simulink library "ESPI_lib"  (Simulink 7.5)
settings: Solver=ode45  StartTime=0.0  StopTime=10.0  RelTol=1e-3
values from neighbouring files (symbols this model uses):
  pESPI_bool_AltitudeSel_C = Simulink.Parameter    [ESPI_par.m]
  pESPI_bool_VehSpdDetdEna_C = Simulink.Parameter    [ESPI_par.m]
  pESPI_kmph_MinSpdSnsrThd_C = Simulink.Parameter    [ESPI_par.m]
  pESPI_kmph_SpdThdPlausibiErr_MAP = Simulink.Parameter    [ESPI_par.m]
  pESPI_kPa_VacAmbPres_C = Simulink.Parameter    [ESPI_par.m]
  pESPI_kPa_VacAmbPres_CUR = Simulink.Parameter    [ESPI_par.m]
  pESPI_m_TireDiam_C = Simulink.Parameter    [ESPI_par.m]
  pESPI_mV_VacAmbPres_TAB = Simulink.Parameter    [ESPI_par.m]
  pESPI_Nm_TrqReqZero_C = Simulink.Parameter    [ESPI_par.m]
  pESPI_pct_ABSFact100_C = Simulink.Parameter    [ESPI_par.m]
  pESPI_ratio_ABSFactRateLo_C = Simulink.Parameter    [ESPI_par.m]
  pESPI_ratio_ABSFactRateUp_C = Simulink.Parameter    [ESPI_par.m]
  pESPI_ratio_AltitudeFacDeflt_C = Simulink.Parameter    [ESPI_par.m]
  pESPI_ratio_AltitudeFacMax_C = Simulink.Parameter    [ESPI_par.m]
  pESPI_ratio_AltitudeFacMin_C = Simulink.Parameter    [ESPI_par.m]
  pESPI_ratio_mpsTokmp_C = Simulink.Parameter    [ESPI_par.m]
  pESPI_ratio_TrsmRat_C = Simulink.Parameter    [ESPI_par.m]
  pESPI_s_NoOfSec_C = Simulink.Parameter    [ESPI_par.m]
undefined symbols (not defined in the file or in its folder): p_bool_False_M, p_bool_True_M, p_single_Minus_M, p_single_Zero_M, VehSpdSourceTyp
libraries: BaseOperationLib_Browser x81, PES_CZ_FAW x6, simulink x1
settings Model: Creator=wuaibin  LastModifiedBy=wuaibin

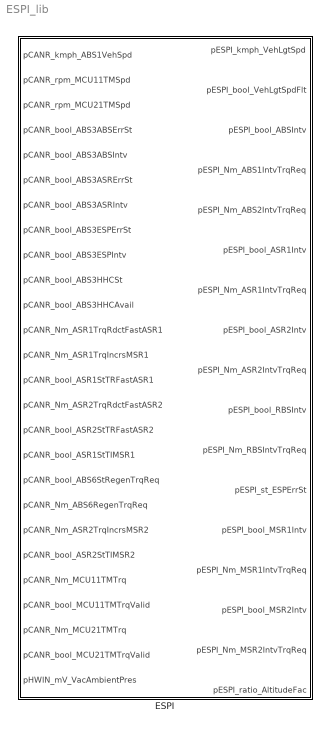
== system ESPI_lib ==
  ESPI : Subsystem  TreatAsAtomicUnit=on

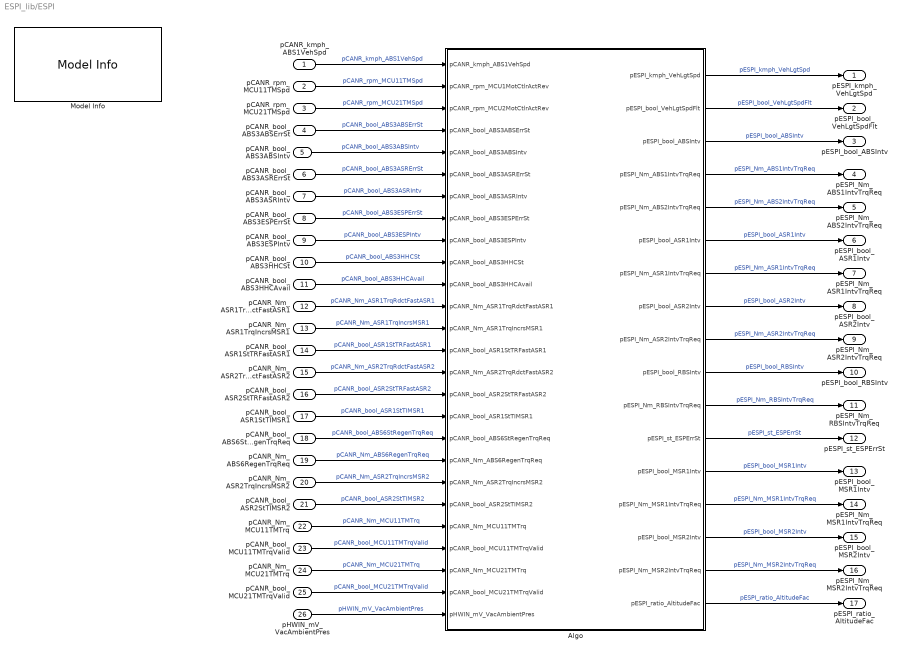
== system ESPI_lib/ESPI ==
  pCANR_kmph_ABS1VehSpd : Inport  OutDataType=fixdt(1, 16)  OutScaling=2^0
  pCANR_rpm_MCU11TMSpd : Inport  Port=2  OutDataType=fixdt(1, 16)  OutScaling=2^0
  pCANR_rpm_MCU21TMSpd : Inport  Port=3  OutDataType=fixdt(1, 16)  OutScaling=2^0
  pCANR_bool_ABS3ABSErrSt : Inport  Port=4  OutDataType=fixdt(1, 16)  OutScaling=2^0
  pCANR_bool_ABS3ABSIntv : Inport  Port=5
  pCANR_bool_ABS3ASRErrSt : Inport  Port=6  OutDataType=fixdt(1, 16)  OutScaling=2^0
  pCANR_bool_ABS3ASRIntv : Inport  Port=7  OutDataType=fixdt(1, 16)  OutScaling=2^0
  pCANR_bool_ABS3ESPErrSt : Inport  Port=8  OutDataType=fixdt(1, 16)  OutScaling=2^0
  pCANR_bool_ABS3ESPIntv : Inport  Port=9  OutDataType=fixdt(1, 16)  OutScaling=2^0
  pCANR_bool_ABS3HHCSt : Inport  Port=10  OutDataType=fixdt(1, 16)  OutScaling=2^0
  pCANR_bool_ABS3HHCAvail : Inport  Port=11  OutDataType=fixdt(1, 16)  OutScaling=2^0
  pCANR_Nm_ASR1TrqRdctFastASR1 : Inport  Port=12  OutDataType=fixdt(1, 16)  OutScaling=2^0
  pCANR_Nm_ASR1TrqIncrsMSR1 : Inport  Port=13  OutDataType=fixdt(1, 16)  OutScaling=2^0
  pCANR_bool_ASR1StTRFastASR1 : Inport  Port=14  OutDataType=fixdt(1, 16)  OutScaling=2^0
  pCANR_Nm_ASR2TrqRdctFastASR2 : Inport  Port=15  OutDataType=fixdt(1, 16)  OutScaling=2^0
  pCANR_bool_ASR2StTRFastASR2 : Inport  Port=16  OutDataType=fixdt(1, 16)  OutScaling=2^0
  pCANR_bool_ASR1StTIMSR1 : Inport  Port=17  OutDataType=fixdt(1, 16)  OutScaling=2^0
  pCANR_bool_ABS6StRegenTrqReq : Inport  Port=18  OutDataType=fixdt(1, 16)  OutScaling=2^0
  pCANR_Nm_ABS6RegenTrqReq : Inport  Port=19  OutDataType=fixdt(1, 16)  OutScaling=2^0
  pCANR_Nm_ASR2TrqIncrsMSR2 : Inport  Port=20  OutDataType=fixdt(1, 16)  OutScaling=2^0
  pCANR_bool_ASR2StTIMSR2 : Inport  Port=21  OutDataType=fixdt(1, 16)  OutScaling=2^0
  pCANR_Nm_MCU11TMTrq : Inport  Port=22
  pCANR_bool_MCU11TMTrqValid : Inport  Port=23
  pCANR_Nm_MCU21TMTrq : Inport  Port=24
  pCANR_bool_MCU21TMTrqValid : Inport  Port=25
  pHWIN_mV_VacAmbientPres : Inport  Port=26
  Algo : Subsystem
  Model Info : simulink/Model-Wide Utilities/Model Info  SystemSampleTime=-1  InitialBlockCM=None  BlockCM=None  Frame=on  DisplayStringWithTags=Model Info\nCreated: %<Created>\nCreator: %<Creator>  HorizontalTextAlignment=Center  LeftAlignmentValue=0.5  SourceBlockDiagram=HQEV_HCU  TagMaxNumber=20
  pESPI_kmph_VehLgtSpd : Outport  OutDataType=fixdt(1, 16)  OutScaling=2^0
  pESPI_bool_VehLgtSpdFlt : Outport  Port=2  OutDataType=fixdt(1, 16)  OutScaling=2^0
  pESPI_bool_ABSIntv : Outport  Port=3  OutDataType=fixdt(1, 16)  OutScaling=2^0
  pESPI_Nm_ABS1IntvTrqReq : Outport  Port=4  OutDataType=fixdt(1, 16)  OutScaling=2^0
  pESPI_Nm_ABS2IntvTrqReq : Outport  Port=5  OutDataType=fixdt(1, 16)  OutScaling=2^0
  pESPI_bool_ASR1Intv : Outport  Port=6  OutDataType=fixdt(1, 16)  OutScaling=2^0
  pESPI_Nm_ASR1IntvTrqReq : Outport  Port=7  OutDataType=fixdt(1, 16)  OutScaling=2^0
  pESPI_bool_ASR2Intv : Outport  Port=8  OutDataType=fixdt(1, 16)  OutScaling=2^0
  pESPI_Nm_ASR2IntvTrqReq : Outport  Port=9  OutDataType=fixdt(1, 16)  OutScaling=2^0
  pESPI_bool_RBSIntv : Outport  Port=10  OutDataType=fixdt(1, 16)  OutScaling=2^0
  pESPI_Nm_RBSIntvTrqReq : Outport  Port=11  OutDataType=fixdt(1, 16)  OutScaling=2^0
  pESPI_st_ESPErrSt : Outport  Port=12  OutDataType=fixdt(1, 16)  OutScaling=2^0
  pESPI_bool_MSR1Intv : Outport  Port=13  OutDataType=fixdt(1, 16)  OutScaling=2^0
  pESPI_Nm_MSR1IntvTrqReq : Outport  Port=14  OutDataType=fixdt(1, 16)  OutScaling=2^0
  pESPI_bool_MSR2Intv : Outport  Port=15  OutDataType=fixdt(1, 16)  OutScaling=2^0
  pESPI_Nm_MSR2IntvTrqReq : Outport  Port=16  OutDataType=fixdt(1, 16)  OutScaling=2^0
  pESPI_ratio_AltitudeFac : Outport  Port=17  OutDataType=fixdt(1, 16)  OutScaling=2^0
  wires:
  pCANR_Nm_MCU11TMTrq/1 -> Algo/22(pCANR_Nm_MCU11TMTrq)  "pCANR_Nm_MCU11TMTrq"
  Algo/5(pESPI_Nm_ABS2IntvTrqReq) -> pESPI_Nm_ABS2IntvTrqReq/1  "pESPI_Nm_ABS2IntvTrqReq"
  pCANR_bool_MCU21TMTrqValid/1 -> Algo/25(pCANR_bool_MCU21TMTrqValid)  "pCANR_bool_MCU21TMTrqValid"
  pCANR_Nm_MCU21TMTrq/1 -> Algo/24(pCANR_Nm_MCU21TMTrq)  "pCANR_Nm_MCU21TMTrq"
  pCANR_bool_MCU11TMTrqValid/1 -> Algo/23(pCANR_bool_MCU11TMTrqValid)  "pCANR_bool_MCU11TMTrqValid"
  Algo/12(pESPI_st_ESPErrSt) -> pESPI_st_ESPErrSt/1  "pESPI_st_ESPErrSt"
  Algo/16(pESPI_Nm_MSR2IntvTrqReq) -> pESPI_Nm_MSR2IntvTrqReq/1  "pESPI_Nm_MSR2IntvTrqReq"
  Algo/15(pESPI_bool_MSR2Intv) -> pESPI_bool_MSR2Intv/1  "pESPI_bool_MSR2Intv"
  Algo/14(pESPI_Nm_MSR1IntvTrqReq) -> pESPI_Nm_MSR1IntvTrqReq/1  "pESPI_Nm_MSR1IntvTrqReq"
  Algo/13(pESPI_bool_MSR1Intv) -> pESPI_bool_MSR1Intv/1  "pESPI_bool_MSR1Intv"
  Algo/8(pESPI_bool_ASR2Intv) -> pESPI_bool_ASR2Intv/1  "pESPI_bool_ASR2Intv"
  Algo/4(pESPI_Nm_ABS1IntvTrqReq) -> pESPI_Nm_ABS1IntvTrqReq/1  "pESPI_Nm_ABS1IntvTrqReq"
  Algo/9(pESPI_Nm_ASR2IntvTrqReq) -> pESPI_Nm_ASR2IntvTrqReq/1  "pESPI_Nm_ASR2IntvTrqReq"
  Algo/11(pESPI_Nm_RBSIntvTrqReq) -> pESPI_Nm_RBSIntvTrqReq/1  "pESPI_Nm_RBSIntvTrqReq"
  Algo/10(pESPI_bool_RBSIntv) -> pESPI_bool_RBSIntv/1  "pESPI_bool_RBSIntv"
  Algo/7(pESPI_Nm_ASR1IntvTrqReq) -> pESPI_Nm_ASR1IntvTrqReq/1  "pESPI_Nm_ASR1IntvTrqReq"
  Algo/6(pESPI_bool_ASR1Intv) -> pESPI_bool_ASR1Intv/1  "pESPI_bool_ASR1Intv"
  Algo/3(pESPI_bool_ABSIntv) -> pESPI_bool_ABSIntv/1  "pESPI_bool_ABSIntv"
  pCANR_bool_ASR2StTIMSR2/1 -> Algo/21(pCANR_bool_ASR2StTIMSR2)  "pCANR_bool_ASR2StTIMSR2"
  pCANR_Nm_ASR2TrqIncrsMSR2/1 -> Algo/20(pCANR_Nm_ASR2TrqIncrsMSR2)  "pCANR_Nm_ASR2TrqIncrsMSR2"
  pCANR_Nm_ABS6RegenTrqReq/1 -> Algo/19(pCANR_Nm_ABS6RegenTrqReq)  "pCANR_Nm_ABS6RegenTrqReq"
  pCANR_bool_ABS6StRegenTrqReq/1 -> Algo/18(pCANR_bool_ABS6StRegenTrqReq)  "pCANR_bool_ABS6StRegenTrqReq"
  pCANR_bool_ASR1StTIMSR1/1 -> Algo/17(pCANR_bool_ASR1StTIMSR1)  "pCANR_bool_ASR1StTIMSR1"
  pCANR_bool_ASR2StTRFastASR2/1 -> Algo/16(pCANR_bool_ASR2StTRFastASR2)  "pCANR_bool_ASR2StTRFastASR2"
  pCANR_Nm_ASR2TrqRdctFastASR2/1 -> Algo/15(pCANR_Nm_ASR2TrqRdctFastASR2)  "pCANR_Nm_ASR2TrqRdctFastASR2"
  pCANR_bool_ASR1StTRFastASR1/1 -> Algo/14(pCANR_bool_ASR1StTRFastASR1)  "pCANR_bool_ASR1StTRFastASR1"
  pCANR_Nm_ASR1TrqIncrsMSR1/1 -> Algo/13(pCANR_Nm_ASR1TrqIncrsMSR1)  "pCANR_Nm_ASR1TrqIncrsMSR1"
  pCANR_Nm_ASR1TrqRdctFastASR1/1 -> Algo/12(pCANR_Nm_ASR1TrqRdctFastASR1)  "pCANR_Nm_ASR1TrqRdctFastASR1"
  pCANR_bool_ABS3HHCAvail/1 -> Algo/11(pCANR_bool_ABS3HHCAvail)  "pCANR_bool_ABS3HHCAvail"
  pCANR_bool_ABS3HHCSt/1 -> Algo/10(pCANR_bool_ABS3HHCSt)  "pCANR_bool_ABS3HHCSt"
  pCANR_bool_ABS3ESPIntv/1 -> Algo/9(pCANR_bool_ABS3ESPIntv)  "pCANR_bool_ABS3ESPIntv"
  pCANR_bool_ABS3ESPErrSt/1 -> Algo/8(pCANR_bool_ABS3ESPErrSt)  "pCANR_bool_ABS3ESPErrSt"
  pCANR_bool_ABS3ASRIntv/1 -> Algo/7(pCANR_bool_ABS3ASRIntv)  "pCANR_bool_ABS3ASRIntv"
  pCANR_bool_ABS3ASRErrSt/1 -> Algo/6(pCANR_bool_ABS3ASRErrSt)  "pCANR_bool_ABS3ASRErrSt"
  pCANR_bool_ABS3ABSIntv/1 -> Algo/5(pCANR_bool_ABS3ABSIntv)  "pCANR_bool_ABS3ABSIntv"
  pCANR_bool_ABS3ABSErrSt/1 -> Algo/4(pCANR_bool_ABS3ABSErrSt)  "pCANR_bool_ABS3ABSErrSt"
  Algo/1(pESPI_kmph_VehLgtSpd) -> pESPI_kmph_VehLgtSpd/1  "pESPI_kmph_VehLgtSpd"
  Algo/2(pESPI_bool_VehLgtSpdFlt) -> pESPI_bool_VehLgtSpdFlt/1  "pESPI_bool_VehLgtSpdFlt"
  pCANR_rpm_MCU21TMSpd/1 -> Algo/3(pCANR_rpm_MCU2MotCtlrActRev)  "pCANR_rpm_MCU21TMSpd"
  pCANR_kmph_ABS1VehSpd/1 -> Algo/1(pCANR_kmph_ABS1VehSpd)  "pCANR_kmph_ABS1VehSpd"
  pCANR_rpm_MCU11TMSpd/1 -> Algo/2(pCANR_rpm_MCU1MotCtlrActRev)  "pCANR_rpm_MCU11TMSpd"
  pHWIN_mV_VacAmbientPres/1 -> Algo/26(pHWIN_mV_VacAmbientPres)  "pHWIN_mV_VacAmbientPres"
  Algo/17(pESPI_ratio_AltitudeFac) -> pESPI_ratio_AltitudeFac/1  "pESPI_ratio_AltitudeFac"

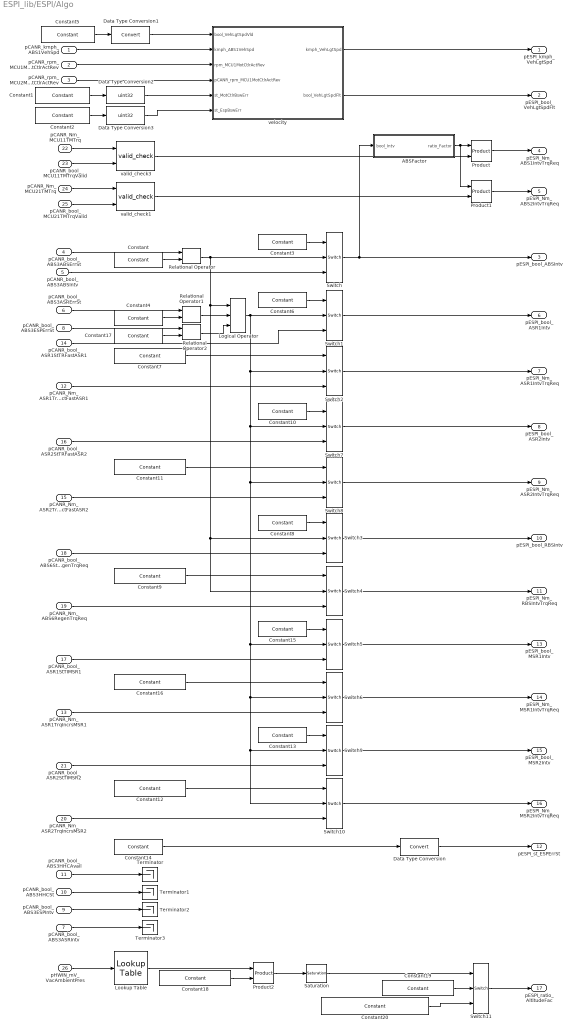
== system ESPI_lib/ESPI/Algo ==
  pCANR_kmph_ABS1VehSpd : Inport  OutDataType=fixdt(1, 16)  OutScaling=2^0
  pCANR_rpm_MCU1MotCtlrActRev : Inport  Port=2  OutDataType=fixdt(1, 16)  OutScaling=2^0
  pCANR_rpm_MCU2MotCtlrActRev : Inport  Port=3  OutDataType=fixdt(1, 16)  OutScaling=2^0
  pCANR_bool_ABS3ABSErrSt : Inport  Port=4  OutDataType=fixdt(1, 16)  OutScaling=2^0
  pCANR_bool_ABS3ABSIntv : Inport  Port=5
  pCANR_bool_ABS3ASRErrSt : Inport  Port=6  OutDataType=fixdt(1, 16)  OutScaling=2^0
  pCANR_bool_ABS3ASRIntv : Inport  Port=7  OutDataType=fixdt(1, 16)  OutScaling=2^0
  pCANR_bool_ABS3ESPErrSt : Inport  Port=8  OutDataType=fixdt(1, 16)  OutScaling=2^0
  pCANR_bool_ABS3ESPIntv : Inport  Port=9  OutDataType=fixdt(1, 16)  OutScaling=2^0
  pCANR_bool_ABS3HHCSt : Inport  Port=10  OutDataType=fixdt(1, 16)  OutScaling=2^0
  pCANR_bool_ABS3HHCAvail : Inport  Port=11  OutDataType=fixdt(1, 16)  OutScaling=2^0
  pCANR_Nm_ASR1TrqRdctFastASR1 : Inport  Port=12  OutDataType=fixdt(1, 16)  OutScaling=2^0
  pCANR_Nm_ASR1TrqIncrsMSR1 : Inport  Port=13  OutDataType=fixdt(1, 16)  OutScaling=2^0
  pCANR_bool_ASR1StTRFastASR1 : Inport  Port=14  OutDataType=fixdt(1, 16)  OutScaling=2^0
  pCANR_Nm_ASR2TrqRdctFastASR2 : Inport  Port=15  OutDataType=fixdt(1, 16)  OutScaling=2^0
  pCANR_bool_ASR2StTRFastASR2 : Inport  Port=16  OutDataType=fixdt(1, 16)  OutScaling=2^0
  pCANR_bool_ASR1StTIMSR1 : Inport  Port=17  OutDataType=fixdt(1, 16)  OutScaling=2^0
  pCANR_bool_ABS6StRegenTrqReq : Inport  Port=18  OutDataType=fixdt(1, 16)  OutScaling=2^0
  pCANR_Nm_ABS6RegenTrqReq : Inport  Port=19  OutDataType=fixdt(1, 16)  OutScaling=2^0
  pCANR_Nm_ASR2TrqIncrsMSR2 : Inport  Port=20  OutDataType=fixdt(1, 16)  OutScaling=2^0
  pCANR_bool_ASR2StTIMSR2 : Inport  Port=21  OutDataType=fixdt(1, 16)  OutScaling=2^0
  pCANR_Nm_MCU11TMTrq : Inport  Port=22
  pCANR_bool_MCU11TMTrqValid : Inport  Port=23
  pCANR_Nm_MCU21TMTrq : Inport  Port=24
  pCANR_bool_MCU21TMTrqValid : Inport  Port=25
  pHWIN_mV_VacAmbientPres : Inport  Port=26
  ABSFactor : Subsystem
  Constant{,4..5,17} (4 alike) : BaseOperationLib_Browser/Sources&Sinks/Constant  Value=p_bool_True_M  OutMin=[]  OutMax=[]  OutDataType=fixdt(1, 16)  ConRadixGroup=Use specified scaling  OutScaling=2^0  OutDataTypeStr=Inherit: Inherit from 'Constant value'
  Constant{1..3,6,8,10,13..15} (9 alike) : BaseOperationLib_Browser/Sources&Sinks/Constant  Value=p_bool_False_M  OutMin=[]  OutMax=[]  OutDataType=fixdt(1, 16)  ConRadixGroup=Use specified scaling  OutScaling=2^0  OutDataTypeStr=Inherit: Inherit from 'Constant value'
  Constant{7,9,11..12,16} (5 alike) : BaseOperationLib_Browser/Sources&Sinks/Constant  Value=pESPI_Nm_TrqReqZero_C  OutMin=[]  OutMax=[]  OutDataType=fixdt(1, 16)  ConRadixGroup=Use specified scaling  OutScaling=2^0  OutDataTypeStr=Inherit: Inherit from 'Constant value'
  Constant18 : BaseOperationLib_Browser/Sources&Sinks/Constant  Value=pESPI_kPa_VacAmbPres_C  OutMin=[]  OutMax=[]  OutDataType=fixdt(1, 16)  ConRadixGroup=Use specified scaling  OutScaling=2^0  OutDataTypeStr=Inherit: Inherit from 'Constant value'
  Constant19 : BaseOperationLib_Browser/Sources&Sinks/Constant  Value=pESPI_bool_AltitudeSel_C  OutMin=[]  OutMax=[]  OutDataType=fixdt(1, 16)  ConRadixGroup=Use specified scaling  OutScaling=2^0  OutDataTypeStr=Inherit: Inherit from 'Constant value'
  Constant20 : BaseOperationLib_Browser/Sources&Sinks/Constant  Value=pESPI_ratio_AltitudeFacDeflt_C  OutMin=[]  OutMax=[]  OutDataType=fixdt(1, 16)  ConRadixGroup=Use specified scaling  OutScaling=2^0  OutDataTypeStr=Inherit: Inherit from 'Constant value'
  Data Type Conversion : DataTypeConversion  OutDataType=fixdt(1, 16)  OutScaling=2^0
  Data Type Conversion1 : DataTypeConversion  OutDataType=fixdt(1, 16)  OutScaling=2^0
  Data Type Conversion2 : DataTypeConversion  OutDataTypeMode=uint32  OutDataType=fixdt(1, 16)  OutScaling=2^0  OutDataTypeStr=uint32
  Data Type Conversion3 : DataTypeConversion  OutDataTypeMode=uint32  OutDataType=fixdt(1, 16)  OutScaling=2^0  OutDataTypeStr=uint32
  Logical Operator : BaseOperationLib_Browser/Logic Operations Changed/Logical Operator  Operator=OR  Inputs=3  AllPortsSameDT=on  OutDataTypeMode=Specify via dialog  LogicDataType=PDT_Bool  OutDataTypeStr=PDT_Bool
  Lookup Table : BaseOperationLib_Browser/Lookup Tables Changed/Lookup Table  InputValues=pESPI_mV_VacAmbPres_TAB  Table=pESPI_kPa_VacAmbPres_CUR  LookUpMeth=Interpolation-Use End Values  OutMin=[]  OutMax=[]  OutDataType=fixdt(1, 16)  OutScaling=2^0  OutDataTypeStr=Inherit: Inherit via back propagation  SaturateOnIntegerOverflow=on
      settings: AttributesFormatString=X:%<InputValues>\nTAB:%<Table>
  Product : BaseOperationLib_Browser/Math Operations Changed/Product  Inputs=2  Multiplication=Element-wise(.*)  OutMin=[]  OutMax=[]  OutDataType=fixdt(1,16,0)  OutScaling=[]  OutDataTypeStr=Inherit: Inherit via back propagation  RndMeth=Zero  SaturateOnIntegerOverflow=on
  Product1 : BaseOperationLib_Browser/Math Operations Changed/Product  Inputs=2  Multiplication=Element-wise(.*)  OutMin=[]  OutMax=[]  OutDataType=fixdt(1,16,0)  OutScaling=[]  OutDataTypeStr=Inherit: Inherit via back propagation  RndMeth=Zero  SaturateOnIntegerOverflow=on
  Product2 : BaseOperationLib_Browser/Math Operations Changed/Product  Inputs=*/  Multiplication=Element-wise(.*)  OutMin=[]  OutMax=[]  OutDataType=fixdt(1,16,0)  OutScaling=[]  OutDataTypeStr=Inherit: Inherit via back propagation  RndMeth=Zero  SaturateOnIntegerOverflow=on
  Relational Operator : BaseOperationLib_Browser/Logic Operations Changed/Relational Operator  Operator===  InputSameDT=on  LogicOutDataTypeMode=Specify via dialog  LogicDataType=PDT_Bool  OutDataTypeStr=PDT_Bool
  Relational Operator1 : BaseOperationLib_Browser/Logic Operations Changed/Relational Operator  Operator===  InputSameDT=on  LogicOutDataTypeMode=Specify via dialog  LogicDataType=PDT_Bool  OutDataTypeStr=PDT_Bool
  Relational Operator2 : BaseOperationLib_Browser/Logic Operations Changed/Relational Operator  Operator===  InputSameDT=on  LogicOutDataTypeMode=Specify via dialog  LogicDataType=PDT_Bool  OutDataTypeStr=PDT_Bool
  Saturation : BaseOperationLib_Browser/Discontinuities Unchanged/Saturation  UpperLimit=pESPI_ratio_AltitudeFacMax_C  LowerLimit=pESPI_ratio_AltitudeFacMin_C  OutMin=[]  OutMax=[]  OutDataType=fixdt(1, 16)  OutScaling=2^0
      settings: AttributesFormatString=ULim:%<UpperLimit>\nLLim:%<LowerLimit>
  Switch{,1..11} (12 alike) : BaseOperationLib_Browser/Signal Routing Changed/Switch  Criteria=u2 ~= 0  Threshold=1  InputSameDT=on  OutMin=[]  OutMax=[]  OutDataType=fixdt(1,16,0)  OutScaling=[]  SaturateOnIntegerOverflow=on
  Terminator{,1..3} (4 alike) : Terminator
  valid_check1 : PES_CZ_FAW/Discontinuities/valid_check  SystemSampleTime=-1  init=0
  valid_check3 : PES_CZ_FAW/Discontinuities/valid_check  SystemSampleTime=-1  init=0
  velocity : Subsystem
  pESPI_kmph_VehLgtSpd : Outport  OutDataType=fixdt(1, 16)  OutScaling=2^0
  pESPI_bool_VehLgtSpdFlt : Outport  Port=2  OutDataType=fixdt(1, 16)  OutScaling=2^0
  pESPI_bool_ABSIntv : Outport  Port=3  OutDataType=fixdt(1, 16)  OutScaling=2^0
  pESPI_Nm_ABS1IntvTrqReq : Outport  Port=4  OutDataType=fixdt(1, 16)  OutScaling=2^0
  pESPI_Nm_ABS2IntvTrqReq : Outport  Port=5  OutDataType=fixdt(1, 16)  OutScaling=2^0
  pESPI_bool_ASR1Intv : Outport  Port=6  OutDataType=fixdt(1, 16)  OutScaling=2^0
  pESPI_Nm_ASR1IntvTrqReq : Outport  Port=7  OutDataType=fixdt(1, 16)  OutScaling=2^0
  pESPI_bool_ASR2Intv : Outport  Port=8  OutDataType=fixdt(1, 16)  OutScaling=2^0
  pESPI_Nm_ASR2IntvTrqReq : Outport  Port=9  OutDataType=fixdt(1, 16)  OutScaling=2^0
  pESPI_bool_RBSIntv : Outport  Port=10  OutDataType=fixdt(1, 16)  OutScaling=2^0
  pESPI_Nm_RBSIntvTrqReq : Outport  Port=11  OutDataType=fixdt(1, 16)  OutScaling=2^0
  pESPI_st_ESPErrSt : Outport  Port=12  OutDataType=fixdt(1, 16)  OutScaling=2^0
  pESPI_bool_MSR1Intv : Outport  Port=13  OutDataType=fixdt(1, 16)  OutScaling=2^0
  pESPI_Nm_MSR1IntvTrqReq : Outport  Port=14  OutDataType=fixdt(1, 16)  OutScaling=2^0
  pESPI_bool_MSR2Intv : Outport  Port=15  OutDataType=fixdt(1, 16)  OutScaling=2^0
  pESPI_Nm_MSR2IntvTrqReq : Outport  Port=16  OutDataType=fixdt(1, 16)  OutScaling=2^0
  pESPI_ratio_AltitudeFac : Outport  Port=17  OutDataType=fixdt(1, 16)  OutScaling=2^0
  wires:
  pCANR_bool_ABS3ESPErrSt/1 -> Relational Operator2/1
  Constant17/1 -> Relational Operator2/2
  Relational Operator2/1 -> Logical Operator/3
  Data Type Conversion/1 -> pESPI_st_ESPErrSt/1
  Product1/1 -> pESPI_Nm_ABS2IntvTrqReq/1
  valid_check1/1 -> Product1/2
  Product/1 -> pESPI_Nm_ABS1IntvTrqReq/1
  valid_check3/1 -> Product/2
  ABSFactor/1(ratio_Factor) -> Product1/1, Product/1
  pCANR_bool_MCU21TMTrqValid/1 -> valid_check1/2
  pCANR_Nm_MCU21TMTrq/1 -> valid_check1/1
  pCANR_bool_MCU11TMTrqValid/1 -> valid_check3/2
  pCANR_Nm_MCU11TMTrq/1 -> valid_check3/1
  Switch9/1 -> pESPI_bool_MSR2Intv/1
  Constant13/1 -> Switch9/1
  Switch10/1 -> pESPI_Nm_MSR2IntvTrqReq/1
  Constant12/1 -> Switch10/1
  pCANR_Nm_ASR2TrqIncrsMSR2/1 -> Switch10/3
  pCANR_bool_ASR2StTIMSR2/1 -> Switch9/3
  Constant11/1 -> Switch8/1
  Switch8/1 -> pESPI_Nm_ASR2IntvTrqReq/1
  pCANR_Nm_ASR2TrqRdctFastASR2/1 -> Switch8/3
  pCANR_bool_ASR2StTRFastASR2/1 -> Switch7/3
  Switch7/1 -> pESPI_bool_ASR2Intv/1
  Constant10/1 -> Switch7/1
  Switch6/1 -> pESPI_Nm_MSR1IntvTrqReq/1
  Constant16/1 -> Switch6/1
  pCANR_Nm_ASR1TrqIncrsMSR1/1 -> Switch6/3
  pCANR_bool_ASR1StTIMSR1/1 -> Switch5/3
  Constant15/1 -> Switch5/1
  Switch5/1 -> pESPI_bool_MSR1Intv/1
  Logical Operator/1 -> Switch8/2, Switch9/2, Switch10/2, Switch6/2, Switch5/2, Switch7/2, Switch2/2, Switch1/2
  Constant14/1 -> Data Type Conversion/1
  pCANR_bool_ABS3ASRIntv/1 -> Terminator3/1
  pCANR_bool_ABS3ESPIntv/1 -> Terminator2/1
  pCANR_bool_ABS3HHCSt/1 -> Terminator1/1
  pCANR_bool_ABS3HHCAvail/1 -> Terminator/1
  Switch4/1 -> pESPI_Nm_RBSIntvTrqReq/1
  pCANR_Nm_ABS6RegenTrqReq/1 -> Switch4/3
  Constant9/1 -> Switch4/1
  Switch3/1 -> pESPI_bool_RBSIntv/1
  Constant8/1 -> Switch3/1
  pCANR_bool_ABS6StRegenTrqReq/1 -> Switch3/3
  Switch2/1 -> pESPI_Nm_ASR1IntvTrqReq/1
  Constant7/1 -> Switch2/1
  pCANR_Nm_ASR1TrqRdctFastASR1/1 -> Switch2/3
  pCANR_bool_ASR1StTRFastASR1/1 -> Switch1/3
  Switch1/1 -> pESPI_bool_ASR1Intv/1
  Switch/1 -> ABSFactor/1(bool_Intv), pESPI_bool_ABSIntv/1
  Constant6/1 -> Switch1/1
  Relational Operator1/1 -> Logical Operator/2
  Constant4/1 -> Relational Operator1/2
  pCANR_bool_ABS3ASRErrSt/1 -> Relational Operator1/1
  pCANR_bool_ABS3ABSIntv/1 -> Switch/3
  Constant3/1 -> Switch/1
  Relational Operator/1 -> Switch4/2, Switch3/2, Logical Operator/1, Switch/2
  Constant/1 -> Relational Operator/2
  pCANR_bool_ABS3ABSErrSt/1 -> Relational Operator/1
  velocity/1(kmph_VehLgtSpd) -> pESPI_kmph_VehLgtSpd/1
  pCANR_kmph_ABS1VehSpd/1 -> velocity/2(kmph_ABS1VehSpd)
  pCANR_rpm_MCU1MotCtlrActRev/1 -> velocity/3(rpm_MCU1MotCtlrActRev)
  velocity/2(bool_VehLgtSpdFlt) -> pESPI_bool_VehLgtSpdFlt/1
  pCANR_rpm_MCU2MotCtlrActRev/1 -> velocity/4(pCANR_rpm_MCU1MotCtlrActRev)
  Constant5/1 -> Data Type Conversion1/1
  Data Type Conversion1/1 -> velocity/1(bool_VehLgtSpdVld)
  Constant1/1 -> Data Type Conversion2/1
  Data Type Conversion2/1 -> velocity/5(st_MotCtlrBswErr)
  Data Type Conversion3/1 -> velocity/6(st_EspBswErr)
  Constant2/1 -> Data Type Conversion3/1
  pHWIN_mV_VacAmbientPres/1 -> Lookup Table/1
  Lookup Table/1 -> Product2/1
  Product2/1 -> Saturation/1
  Constant18/1 -> Product2/2
  Saturation/1 -> Switch11/1
  Switch11/1 -> pESPI_ratio_AltitudeFac/1
  Constant19/1 -> Switch11/2
  Constant20/1 -> Switch11/3

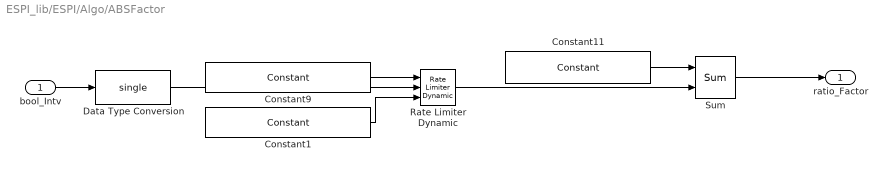
== system ESPI_lib/ESPI/Algo/ABSFactor ==
  bool_Intv : Inport  OutDataType=fixdt(1, 16)  OutScaling=2^0
  Constant1 : BaseOperationLib_Browser/Sources&Sinks/Constant  Value=pESPI_ratio_ABSFactRateLo_C  OutMin=[]  OutMax=[]  OutDataType=fixdt(1, 16)  ConRadixGroup=Use specified scaling  OutScaling=2^0  OutDataTypeStr=Inherit: Inherit from 'Constant value'
  Constant11 : BaseOperationLib_Browser/Sources&Sinks/Constant  Value=pESPI_pct_ABSFact100_C  OutMin=[]  OutMax=[]  OutDataType=fixdt(1, 16)  ConRadixGroup=Use specified scaling  OutScaling=2^0  OutDataTypeStr=Inherit: Inherit from 'Constant value'
  Constant9 : BaseOperationLib_Browser/Sources&Sinks/Constant  Value=pESPI_ratio_ABSFactRateUp_C  OutMin=[]  OutMax=[]  OutDataType=fixdt(1, 16)  ConRadixGroup=Use specified scaling  OutScaling=2^0  OutDataTypeStr=Inherit: Inherit from 'Constant value'
  Data Type Conversion : DataTypeConversion  OutDataTypeMode=single  OutDataType=fixdt(1, 16)  OutScaling=2^0  OutDataTypeStr=single
  Rate Limiter Dynamic : BaseOperationLib_Browser/Discontinuities Unchanged/Rate Limiter Dynamic  SystemSampleTime=-1
  Sum : BaseOperationLib_Browser/Math Operations Changed/Sum  Inputs=+-  InputSameDT=on  OutMin=[]  OutMax=[]  OutDataType=fixdt(1, 16)  OutScaling=2^0  SaturateOnIntegerOverflow=on
  ratio_Factor : Outport  OutDataType=fixdt(1, 16)  OutScaling=2^0
  wires:
  bool_Intv/1 -> Data Type Conversion/1
  Sum/1 -> ratio_Factor/1
  Data Type Conversion/1 -> Rate Limiter Dynamic/2
  Constant9/1 -> Rate Limiter Dynamic/1
  Constant1/1 -> Rate Limiter Dynamic/3
  Rate Limiter Dynamic/1 -> Sum/2
  Constant11/1 -> Sum/1

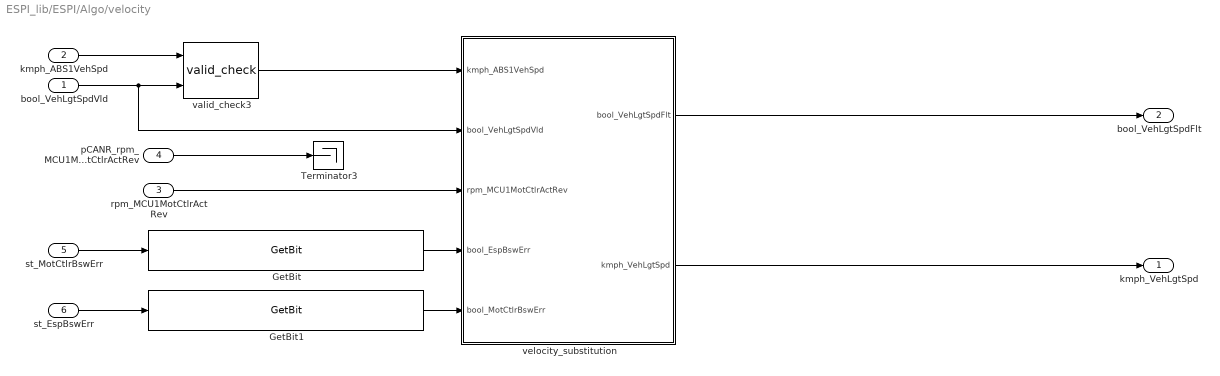
== system ESPI_lib/ESPI/Algo/velocity ==
  bool_VehLgtSpdVld : Inport  OutDataType=fixdt(1, 16)  OutScaling=2^0
  kmph_ABS1VehSpd : Inport  Port=2  OutDataType=fixdt(1, 16)  OutScaling=2^0
  rpm_MCU1MotCtlrActRev : Inport  Port=3  OutDataType=fixdt(1, 16)  OutScaling=2^0
  pCANR_rpm_MCU1MotCtlrActRev : Inport  Port=4  OutDataType=fixdt(1, 16)  OutScaling=2^0
  st_MotCtlrBswErr : Inport  Port=5  OutDataType=fixdt(1, 16)  OutScaling=2^0
  st_EspBswErr : Inport  Port=6  OutDataType=fixdt(1, 16)  OutScaling=2^0
  GetBit : PES_CZ_FAW/Discontinuities/GetBit  SystemSampleTime=-1  maska=FAWMotCtlrBswErrTyp.MCU1_COMMUNICATION_ERROR
  GetBit1 : PES_CZ_FAW/Discontinuities/GetBit  SystemSampleTime=-1  maska=FAWEspBswErrTyp.ABS1_COMMUNICATION_ERROR
  Terminator3 : Terminator
  valid_check3 : PES_CZ_FAW/Discontinuities/valid_check  SystemSampleTime=-1  init=0
  velocity_substitution : Subsystem
  kmph_VehLgtSpd : Outport  OutDataType=fixdt(1, 16)  OutScaling=2^0
  bool_VehLgtSpdFlt : Outport  Port=2  OutDataType=fixdt(1, 16)  OutScaling=2^0
  wires:
  pCANR_rpm_MCU1MotCtlrActRev/1 -> Terminator3/1
  velocity_substitution/1(bool_VehLgtSpdFlt) -> bool_VehLgtSpdFlt/1
  velocity_substitution/2(kmph_VehLgtSpd) -> kmph_VehLgtSpd/1
  bool_VehLgtSpdVld/1 -> valid_check3/2, velocity_substitution/2(bool_VehLgtSpdVld)
  kmph_ABS1VehSpd/1 -> valid_check3/1
  rpm_MCU1MotCtlrActRev/1 -> velocity_substitution/3(rpm_MCU1MotCtlrActRev)
  valid_check3/1 -> velocity_substitution/1(kmph_ABS1VehSpd)
  st_MotCtlrBswErr/1 -> GetBit/1
  st_EspBswErr/1 -> GetBit1/1
  GetBit/1 -> velocity_substitution/4(bool_EspBswErr)
  GetBit1/1 -> velocity_substitution/5(bool_MotCtlrBswErr)

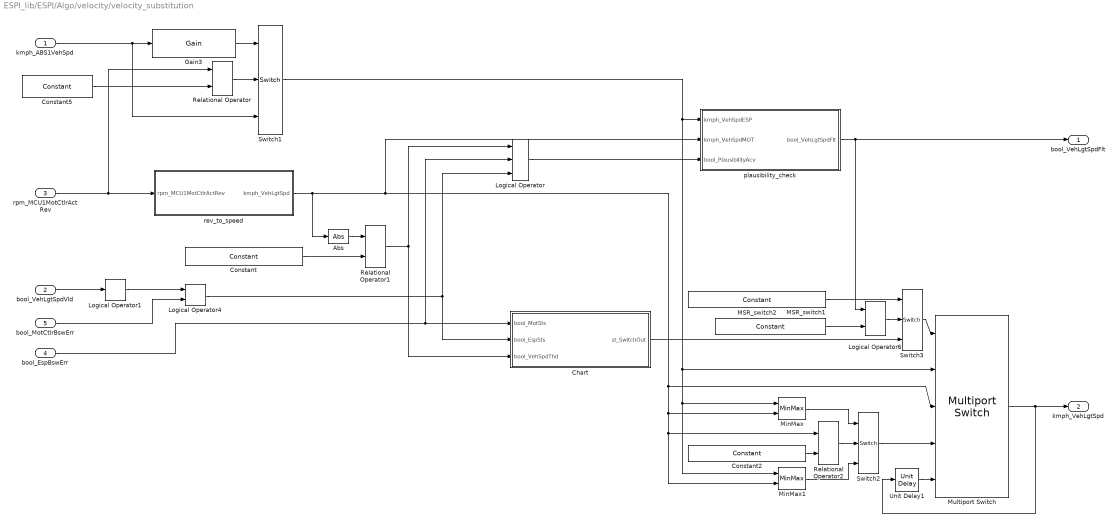
== system ESPI_lib/ESPI/Algo/velocity/velocity_substitution ==
  kmph_ABS1VehSpd : Inport
  bool_VehLgtSpdVld : Inport  Port=2
  rpm_MCU1MotCtlrActRev : Inport  Port=3
  bool_EspBswErr : Inport  Port=4
  bool_MotCtlrBswErr : Inport  Port=5
  Abs : BaseOperationLib_Browser/Math Operations Changed/Abs  OutMax=[]  OutDataType=fixdt(1, 16)  OutScaling=2^0  SaturateOnIntegerOverflow=on
  Chart : Stateflow chart  TreatAsAtomicUnit=on
  Constant : BaseOperationLib_Browser/Sources&Sinks/Constant  Value=pESPI_kmph_MinSpdSnsrThd_C  OutMin=[]  OutMax=[]  OutDataType=fixdt(1, 16)  ConRadixGroup=Use specified scaling  OutScaling=2^0  OutDataTypeStr=Inherit: Inherit from 'Constant value'
  Constant2 : BaseOperationLib_Browser/Sources&Sinks/Constant  Value=pESPI_kmph_MinSpdSnsrThd_C  OutMin=[]  OutMax=[]  OutDataType=fixdt(1, 16)  ConRadixGroup=Use specified scaling  OutScaling=2^0  OutDataTypeStr=Inherit: Inherit from 'Constant value'
  Constant5 : BaseOperationLib_Browser/Sources&Sinks/Constant  Value=p_single_Zero_M  OutMin=[]  OutMax=[]  OutDataType=fixdt(1, 16)  ConRadixGroup=Use specified scaling  OutScaling=2^0  OutDataTypeStr=Inherit: Inherit from 'Constant value'
  Gain3 : BaseOperationLib_Browser/Math Operations Changed/Gain  Gain=p_single_Minus_M  Multiplication=Element-wise(K.*u)  ParamMin=[]  ParamMax=[]  ParameterDataType=fixdt(1, 16)  ParameterScalingMode=Best Precision: Matrix-wise  ParameterScaling=2^0  ParamDataTypeStr=Inherit: Inherit from 'Gain'  OutMin=[]  OutMax=[]  OutDataType=fixdt(1, 16)  OutScaling=2^0  SaturateOnIntegerOverflow=on
  Logical Operator : BaseOperationLib_Browser/Logic Operations Changed/Logical Operator  Operator=NOR  Inputs=3  AllPortsSameDT=on  OutDataTypeMode=Specify via dialog  LogicDataType=PDT_Bool  OutDataTypeStr=PDT_Bool
  Logical Operator1 : BaseOperationLib_Browser/Logic Operations Changed/Logical Operator  Operator=NOT  Inputs=3  AllPortsSameDT=on  OutDataTypeMode=Specify via dialog  LogicDataType=PDT_Bool  OutDataTypeStr=PDT_Bool
  Logical Operator4 : BaseOperationLib_Browser/Logic Operations Changed/Logical Operator  Operator=OR  Inputs=2  AllPortsSameDT=on  OutDataTypeMode=Specify via dialog  LogicDataType=PDT_Bool  OutDataTypeStr=PDT_Bool
  Logical Operator6 : BaseOperationLib_Browser/Logic Operations Changed/Logical Operator  Operator=AND  Inputs=2  AllPortsSameDT=on  OutDataTypeMode=Specify via dialog  LogicDataType=PDT_Bool  OutDataTypeStr=PDT_Bool
  MSR_switch1 : BaseOperationLib_Browser/Sources&Sinks/Constant  Value=pESPI_bool_VehSpdDetdEna_C  OutMin=[]  OutMax=[]  OutDataTypeMode=boolean  OutDataType=fixdt(1, 16)  ConRadixGroup=Use specified scaling  OutScaling=2^0  OutDataTypeStr=boolean
  MSR_switch2 : BaseOperationLib_Browser/Sources&Sinks/Constant  Value=uint8(VehSpdSourceTyp.SPD_PLAUSI)  OutMin=[]  OutMax=[]  OutDataType=Enum: VehSpdSourceTyp  ConRadixGroup=Best Precision: Vector-wise  OutScaling=[]  OutDataTypeStr=Inherit: Inherit from 'Constant value'
  MinMax : BaseOperationLib_Browser/Math Operations Changed/MinMax  Function=max  Inputs=2  InputSameDT=on  OutMin=[]  OutMax=[]  OutDataType=fixdt(1, 16)  OutScaling=2^0  SaturateOnIntegerOverflow=on
  MinMax1 : BaseOperationLib_Browser/Math Operations Changed/MinMax  Function=min  Inputs=2  InputSameDT=on  OutMin=[]  OutMax=[]  OutDataType=fixdt(1, 16)  OutScaling=2^0  SaturateOnIntegerOverflow=on
  Multiport Switch : BaseOperationLib_Browser/Signal Routing Changed/Multiport Switch  DataPortOrder=Specify indices  Inputs=4  DataPortIndices={uint8(VehSpdSourceTyp.SPD_ESP),uint8(VehSpdSourceTyp.SPD_MOTOR),uint8(VehSpdSourceTyp.SPD_PLAUSI),uint8(VehSpdSourceTyp.SPD_SUBS)}  zeroidx=off  InputSameDT=on  OutMin=[]  OutMax=[]  OutDataType=fixdt(1, 16)  OutScaling=2^0  SaturateOnIntegerOverflow=on
  Relational Operator : BaseOperationLib_Browser/Logic Operations Changed/Relational Operator  Operator=<  InputSameDT=on  LogicOutDataTypeMode=Specify via dialog  LogicDataType=PDT_Bool  OutDataTypeStr=PDT_Bool
  Relational Operator1 : BaseOperationLib_Browser/Logic Operations Changed/Relational Operator  Operator=<=  InputSameDT=on  LogicOutDataTypeMode=Specify via dialog  LogicDataType=PDT_Bool  OutDataTypeStr=PDT_Bool
  Relational Operator2 : BaseOperationLib_Browser/Logic Operations Changed/Relational Operator  Operator=>=  InputSameDT=on  LogicOutDataTypeMode=Specify via dialog  LogicDataType=PDT_Bool  OutDataTypeStr=PDT_Bool
  Switch1 : BaseOperationLib_Browser/Signal Routing Changed/Switch  Criteria=u2 ~= 0  Threshold=1  InputSameDT=on  OutMin=[]  OutMax=[]  OutDataType=fixdt(1,16,0)  OutScaling=[]  SaturateOnIntegerOverflow=on
  Switch2 : BaseOperationLib_Browser/Signal Routing Changed/Switch  Criteria=u2 ~= 0  Threshold=1  InputSameDT=on  OutMin=[]  OutMax=[]  OutDataType=fixdt(1,16,0)  OutScaling=[]  SaturateOnIntegerOverflow=on
  Switch3 : BaseOperationLib_Browser/Signal Routing Changed/Switch  Criteria=u2 ~= 0  Threshold=1  InputSameDT=on  OutMin=[]  OutMax=[]  OutDataType=fixdt(1,16,0)  OutScaling=[]  SaturateOnIntegerOverflow=on
  Unit Delay1 : BaseOperationLib_Browser/Discrete Unchanged /Unit Delay  X0=0  SampleTime=-1
  plausibility_check : Subsystem
  rev_to_speed : Subsystem
  bool_VehLgtSpdFlt : Outport
  kmph_VehLgtSpd : Outport  Port=2
  wires:
  Chart/1(st_SwitchOut) -> Switch3/3
  MSR_switch2/1 -> Switch3/1
  Switch3/1 -> Multiport Switch/1
  Unit Delay1/1 -> Multiport Switch/5
  Multiport Switch/1 -> kmph_VehLgtSpd/1, Unit Delay1/1
  MSR_switch1/1 -> Logical Operator6/2
  Logical Operator6/1 -> Switch3/2
  Constant2/1 -> Relational Operator2/2
  Relational Operator2/1 -> Switch2/2
  Switch2/1 -> Multiport Switch/4
  MinMax/1 -> Switch2/1
  MinMax1/1 -> Switch2/3
  plausibility_check/1(bool_VehLgtSpdFlt) -> Logical Operator6/1, bool_VehLgtSpdFlt/1
  rev_to_speed/1(kmph_VehLgtSpd) -> Multiport Switch/3, MinMax/2, Relational Operator2/1, MinMax1/2, plausibility_check/2(kmph_VehSpdMOT), Abs/1
  Relational Operator1/1 -> Chart/3(bool_VehSpdThd), Logical Operator/1
  Abs/1 -> Relational Operator1/1
  rpm_MCU1MotCtlrActRev/1 -> rev_to_speed/1(rpm_MCU1MotCtlrActRev), Relational Operator/1
  kmph_ABS1VehSpd/1 -> Gain3/1, Switch1/3
  Relational Operator/1 -> Switch1/2
  Gain3/1 -> Switch1/1
  Switch1/1 -> Multiport Switch/2, MinMax/1, MinMax1/1, plausibility_check/1(kmph_VehSpdESP)
  Constant5/1 -> Relational Operator/2
  Constant/1 -> Relational Operator1/2
  bool_VehLgtSpdVld/1 -> Logical Operator1/1
  Logical Operator/1 -> plausibility_check/3(bool_PlausibilityAcv)
  Logical Operator1/1 -> Logical Operator4/1
  Logical Operator4/1 -> Logical Operator/3, Chart/2(bool_EspSts)
  bool_EspBswErr/1 -> Logical Operator/2, Chart/1(bool_MotSts)
  bool_MotCtlrBswErr/1 -> Logical Operator4/2

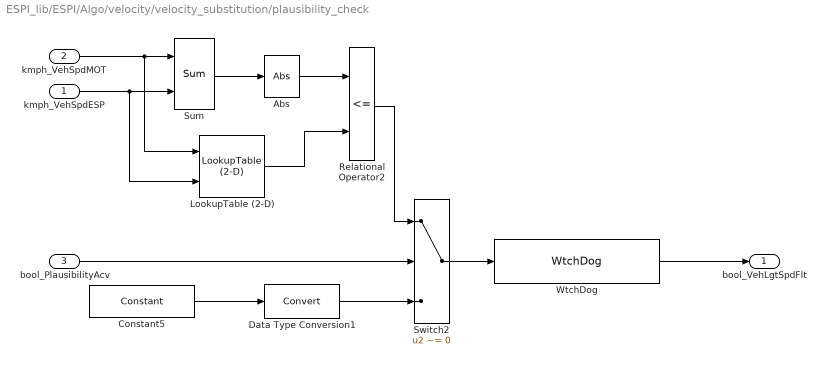
== system ESPI_lib/ESPI/Algo/velocity/velocity_substitution/plausibility_check ==
  kmph_VehSpdESP : Inport
  kmph_VehSpdMOT : Inport  Port=2
  bool_PlausibilityAcv : Inport  Port=3
  Abs : BaseOperationLib_Browser/Math Operations Changed/Abs  OutMax=[]  OutDataType=fixdt(1, 16)  OutScaling=2^0  SaturateOnIntegerOverflow=on
  Constant5 : BaseOperationLib_Browser/Sources&Sinks/Constant  Value=p_bool_True_M  OutMin=[]  OutMax=[]  OutDataType=fixdt(1, 16)  ConRadixGroup=Use specified scaling  OutScaling=2^0  OutDataTypeStr=Inherit: Inherit from 'Constant value'
  Data Type Conversion1 : DataTypeConversion  OutDataType=fixdt(1, 16)  OutScaling=2^0
  LookupTable (2-D) : BaseOperationLib_Browser/Lookup Tables Changed/LookupTable (2-D)  RowIndex=pESPI_kmph_VehSpdMot_TABX  ColumnIndex=pESPI_kmph_VehSpdEsp_TABY  Table=pESPI_kmph_SpdThdPlausibiErr_MAP  LookUpMeth=Interpolation-Use End Values  OutMin=[]  OutMax=[]  OutDataType=fixdt(1, 16)  OutScaling=2^0  OutDataTypeStr=Inherit: Inherit via back propagation  SaturateOnIntegerOverflow=on
      settings: AttributesFormatString=X:%<RowIndex>\nY:%<ColumnIndex>\nTAB:%<Table>
  Relational Operator2 : RelationalOperator  Operator=<=  LogicOutDataTypeMode=Specify via dialog  LogicDataType=PDT_Bool  OutDataTypeStr=PDT_Bool  InputSameDT=on
      mask Display: patch([0 1 1 1 .75], [1 1 0 .75 1], [0 1 0]);
  Sum : BaseOperationLib_Browser/Math Operations Changed/Sum  Inputs=+-  InputSameDT=on  OutMin=[]  OutMax=[]  OutDataType=fixdt(1, 16)  OutScaling=2^0  SaturateOnIntegerOverflow=on
  Switch2 : Switch  Criteria=u2 ~= 0
      mask Display: patch([0 1 1 1 .75], [1 1 0 .75 1], [0 1 0]);
  WtchDog : PES_CZ_FAW/Discontinuities/WtchDog  SystemSampleTime=-1  timeoutthres=pESPI_s_TiDlyVehSpdP_C
  bool_VehLgtSpdFlt : Outport
  wires:
  Data Type Conversion1/1 -> Switch2/3
  Switch2/1 -> WtchDog/1
  Relational Operator2/1 -> Switch2/1
  LookupTable (2-D)/1 -> Relational Operator2/2
  Sum/1 -> Abs/1
  Constant5/1 -> Data Type Conversion1/1
  kmph_VehSpdMOT/1 -> Sum/1, LookupTable (2-D)/1
  kmph_VehSpdESP/1 -> Sum/2, LookupTable (2-D)/2
  bool_PlausibilityAcv/1 -> Switch2/2
  WtchDog/1 -> bool_VehLgtSpdFlt/1
  Abs/1 -> Relational Operator2/1

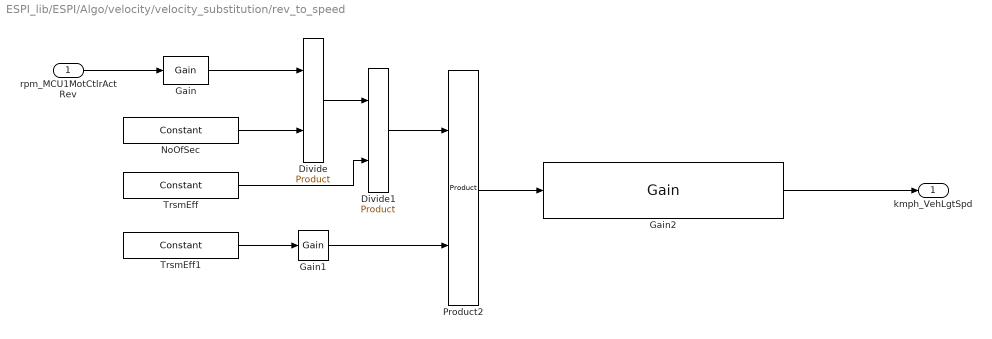
== system ESPI_lib/ESPI/Algo/velocity/velocity_substitution/rev_to_speed ==
  rpm_MCU1MotCtlrActRev : Inport
  Divide : BaseOperationLib_Browser/Math Operations Changed/Product  Inputs=*/  Multiplication=Element-wise(.*)  OutMin=[]  OutMax=[]  OutDataType=fixdt(1,16,0)  OutScaling=[]
  Divide1 : BaseOperationLib_Browser/Math Operations Changed/Product  Inputs=*/  Multiplication=Element-wise(.*)  OutMin=[]  OutMax=[]  OutDataType=fixdt(1,16,0)  OutScaling=[]
  Gain : BaseOperationLib_Browser/Math Operations Changed/Gain  Gain=2*pi  Multiplication=Element-wise(K.*u)  ParamMin=[]  ParamMax=[]  ParameterDataType=fixdt(1, 16)  ParameterScalingMode=Best Precision: Matrix-wise  ParameterScaling=2^0  OutMin=[]  OutMax=[]  OutDataType=fixdt(1, 16)  OutScaling=2^0
  Gain1 : BaseOperationLib_Browser/Math Operations Changed/Gain  Gain=1/2  Multiplication=Element-wise(K.*u)  ParamMin=[]  ParamMax=[]  ParameterDataType=fixdt(1, 16)  ParameterScalingMode=Best Precision: Matrix-wise  ParameterScaling=2^0  OutMin=[]  OutMax=[]  OutDataType=fixdt(1, 16)  OutScaling=2^0
  Gain2 : BaseOperationLib_Browser/Math Operations Changed/Gain  Gain=pESPI_ratio_mpsTokmp_C  Multiplication=Element-wise(K.*u)  ParamMin=[]  ParamMax=[]  ParameterDataType=fixdt(1, 16)  ParameterScalingMode=Best Precision: Matrix-wise  ParameterScaling=2^0  OutMin=[]  OutMax=[]  OutDataType=fixdt(1, 16)  OutScaling=2^0
  NoOfSec : BaseOperationLib_Browser/Sources&Sinks/Constant  Value=pESPI_s_NoOfSec_C  OutMin=[]  OutMax=[]  OutDataTypeMode=single  OutDataType=fixdt(1, 16)  ConRadixGroup=Use specified scaling  OutScaling=2^0  OutDataTypeStr=single
  Product2 : BaseOperationLib_Browser/Math Operations Changed/Product  Inputs=2  Multiplication=Element-wise(.*)  OutMin=[]  OutMax=[]  OutDataType=fixdt(1,16,0)  OutScaling=[]  RndMeth=Zero
  TrsmEff : BaseOperationLib_Browser/Sources&Sinks/Constant  Value=pESPI_ratio_TrsmRat_C  OutMin=[]  OutMax=[]  OutDataTypeMode=single  OutDataType=fixdt(1, 16)  ConRadixGroup=Use specified scaling  OutScaling=2^0  OutDataTypeStr=single
  TrsmEff1 : BaseOperationLib_Browser/Sources&Sinks/Constant  Value=pESPI_m_TireDiam_C  OutMin=[]  OutMax=[]  OutDataTypeMode=single  OutDataType=fixdt(1, 16)  ConRadixGroup=Use specified scaling  OutScaling=2^0  OutDataTypeStr=single
  kmph_VehLgtSpd : Outport
  wires:
  Divide1/1 -> Product2/1
  Divide/1 -> Divide1/1
  Gain2/1 -> kmph_VehLgtSpd/1
  rpm_MCU1MotCtlrActRev/1 -> Gain/1
  TrsmEff1/1 -> Gain1/1
  Gain1/1 -> Product2/2
  Gain/1 -> Divide/1
  NoOfSec/1 -> Divide/2
  TrsmEff/1 -> Divide1/2
  Product2/1 -> Gain2/1

== stateflow chart ESPI/Algo/velocity/velocity_substitution/Chart ==
  state Normal
    state SPD_SUBS
      en:
      st_SwitchOut = VehSpdSourceTyp.SPD_SUBS;
    state SPD_ESP
      du:
      st_SwitchOut = VehSpdSourceTyp.SPD_ESP;
    state SPD_MOTOR
      du:
      st_SwitchOut = VehSpdSourceTyp.SPD_MOTOR;
    (default) -> SPD_SUBS
    SPD_SUBS -> SPD_ESP [order 2] : [bool_MotSts]
    SPD_SUBS -> SPD_MOTOR [order 1] : [bool_VehSpdThd && ...
        | (!bool_MotSts && ...
        | !bool_EspSts) || ...
        | (bool_EspSts && ...
        | !bool_MotSts)]
    SPD_ESP -> SPD_MOTOR : [bool_EspSts || ...
        | (bool_VehSpdThd && ...
        | !bool_MotSts)]
    SPD_MOTOR -> SPD_ESP : [(!bool_VehSpdThd && ...
        | !bool_EspSts) || ...
        | bool_MotSts]
  state Error
    en:
    st_SwitchOut = VehSpdSourceTyp.SPD_ESP;
  (default) -> Normal
  Normal -> Error : [bool_MotSts && ...
      | bool_EspSts]
  Error -> Normal : [!bool_MotSts || ...
      | !bool_EspSts]
  data: st_SwitchOut output uint8; bool_MotSts input double; bool_EspSts input double; bool_VehSpdThd input double
